simulink model "VTOL_thrust_representation_descent"  (R2020b)
settings: Solver=VariableStepAuto  StartTime=0.0  StopTime=60  RelTol=1e-3
values from neighbouring files (symbols this model uses):
  Aproj = 8.8    [Descent_VTOL_Controller_Design.m]
  Cdvertical = 1    [Descent_VTOL_Controller_Design.m]
  g = 32    [Descent_VTOL_Controller_Design.m]
  Ixx = 13900*lbm2slug/144    (= 2.99236111111)    [Descent_VTOL_Controller_Design.m]
  Ixy = -220*lbm2slug/144    (= -0.0473611111111)    [Descent_VTOL_Controller_Design.m]
  Ixz = -720*lbm2slug/144    (= -0.155)    [Descent_VTOL_Controller_Design.m]
  Iyy = 20150*lbm2slug/144    (= 4.33784722222)    [Descent_VTOL_Controller_Design.m]
  Iyz = -1271*lbm2slug/144    (= -0.273618055556)    [Descent_VTOL_Controller_Design.m]
  Izz = 8300*lbm2slug/144    (= 1.78680555556)    [Descent_VTOL_Controller_Design.m]
  K = lqr(A,B,Q,R)    [Descent_VTOL_Controller_Design.m]
  m = 120*lbm2slug    (= 3.72)    [Descent_VTOL_Controller_Design.m]
  rho = 0.0024    [Descent_VTOL_Controller_Design.m]
  Tbig = 56    [Descent_VTOL_Controller_Design.m]
  Tsmall = 33    [Descent_VTOL_Controller_Design.m]
  xcg1 = (37 - 13.6)/12    (= 1.95)    [Descent_VTOL_Controller_Design.m]
  xcg2 = (44.25 - 37)/12    (= 0.604166666667)    [Descent_VTOL_Controller_Design.m]
undefined symbols (not defined in the file or in its folder): magnitude
libraries: simulink x4, shared6dof x1, aerolibanim x1, dspsigops x1
settings Model: Creator=natha  LastModifiedBy=natha

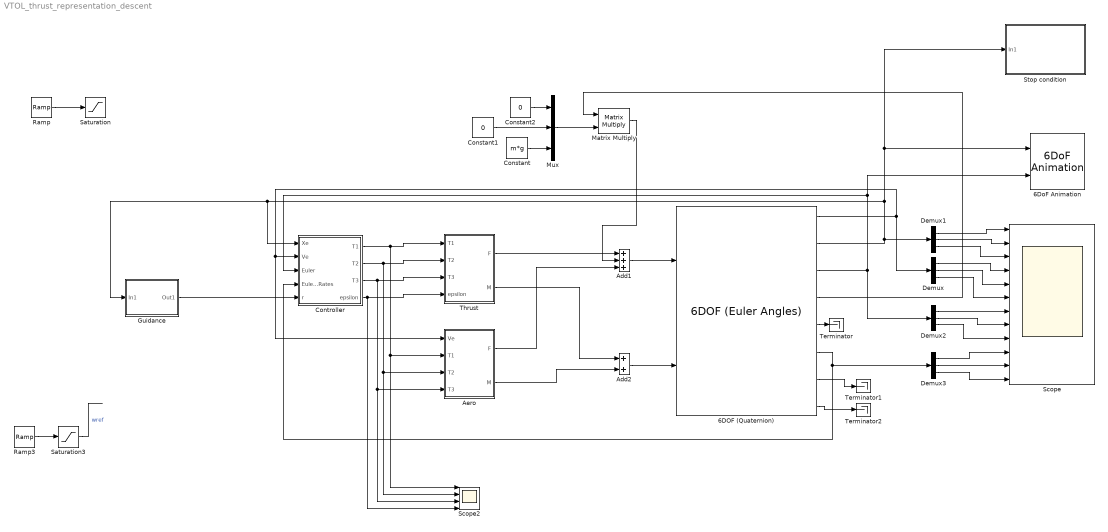
== system VTOL_thrust_representation_descent ==
  6DOF (Quaternion) : shared6dof/6DOF (Euler Angles)  units=Metric (MKS)  mtype=Fixed  rep=Quaternion  xme_0=[0 0 -100]  Vm_0=[0 0 3]  eul_0=[0 0 0]  pm_0=[0 0 0]  mass_0=m  mass_e=0.5  mass_f=2.0  inertia=[Ixx Ixy Ixz; Ixy Iyy Iyz; Ixz Iyz Izz]  inertia_e=eye(3)  inertia_f=2*eye(3)  k_quat=1.0  vre_flag=on  abi_flag=off  aMode=0  xme_statename=''  Vm_statename=''  eul_statename=''  quat_statename=''  pm_statename=''  mass_statename=''
      settings: SourceProductBaseCode=AE,PW,MT,UV,VE,VP
  6DoF Animation : aerolibanim/6DoF Animation  u1=[0 4000 -200 200 -200 200]  u2=0.1  u3=4  u4=[0 0 0]  u5=Fly alongside  u6=[30 100 -30]  u7=10  u8=on
  Add1 : Sum  Inputs=+++
  Add2 : Sum
  Aero : Subsystem
  Constant : Constant  Value=m*g
  Constant1 : Constant  Value=0
  Constant2 : Constant  Value=0
  Controller : Subsystem
  Demux{,1..3} (4 alike) : Demux  Outputs=3
  Guidance : Subsystem
  Matrix Multiply : Product  Multiplication=Matrix(*)
  Mux : Mux  Inputs=3
  Ramp : simulink/Sources/Ramp  slope=-2  start=0  InitialOutput=0
  Ramp3 : simulink/Sources/Ramp  slope=-1  start=0  InitialOutput=0
  Saturation : Saturate  UpperLimit=0  LowerLimit=-5  LinearizeAsGain=off
  Saturation3 : Saturate  UpperLimit=3  LowerLimit=0.5  LinearizeAsGain=off
  Scope : Scope  NumInputPorts=12
  Scope2 : Scope  NumInputPorts=4
  Stop condition : Subsystem
  Terminator : Terminator
  Terminator1 : Terminator
  Terminator2 : Terminator
  Thrust : Subsystem
  wires:
  Demux/2 -> Scope/5
  Demux2/3 -> Scope/9
  Demux3/1 -> Scope/10
  Demux/1 -> Scope/4
  Demux2/2 -> Scope/8
  Demux1/2 -> Scope/2
  Demux1/1 -> Scope/1
  Thrust/1(F) -> Add1/1
  Constant1/1 -> Mux/2
  Matrix Multiply/1 -> Add1/2
  Mux/1 -> Matrix Multiply/2
  Add1/1 -> 6DOF (Quaternion)/1
  Demux/3 -> Scope/6
  6DOF (Quaternion)/3 -> Demux2/1, 6DoF Animation/2, Controller/3(Euler)
  6DOF (Quaternion)/1 -> Demux/1, Aero/1(Ve), Controller/2(Ve)
  Demux3/3 -> Scope/12
  Demux2/1 -> Scope/7
  6DOF (Quaternion)/4 -> Matrix Multiply/1
  6DOF (Quaternion)/2 -> Demux1/1, Stop condition/1(In1), 6DoF Animation/1, Guidance/1(In1), Controller/1(Xe)
  Demux1/3 -> Scope/3
  Demux3/2 -> Scope/11
  Constant2/1 -> Mux/1
  Constant/1 -> Mux/3
  6DOF (Quaternion)/6 -> Demux3/1, Controller/4(Euler Rates)
  Controller/4(epsilon) -> Thrust/4(epsilon), Scope2/4
  Controller/2(T2) -> Aero/3(T2), Scope2/2, Thrust/2(T2)
  Controller/3(T3) -> Aero/4(T3), Scope2/3, Thrust/3(T3)
  Controller/1(T1) -> Aero/2(T1), Scope2/1, Thrust/1(T1)
  Add2/1 -> 6DOF (Quaternion)/2
  Aero/2(M) -> Add2/2
  Thrust/2(M) -> Add2/1
  Aero/1(F) -> Add1/3
  Ramp/1 -> Saturation/1
  6DOF (Quaternion)/5 -> Terminator/1
  6DOF (Quaternion)/7 -> Terminator1/1
  6DOF (Quaternion)/8 -> Terminator2/1
  Ramp3/1 -> Saturation3/1
  Saturation3/1 -> ?  "wref"
  Guidance/1(Out1) -> Controller/5(r)

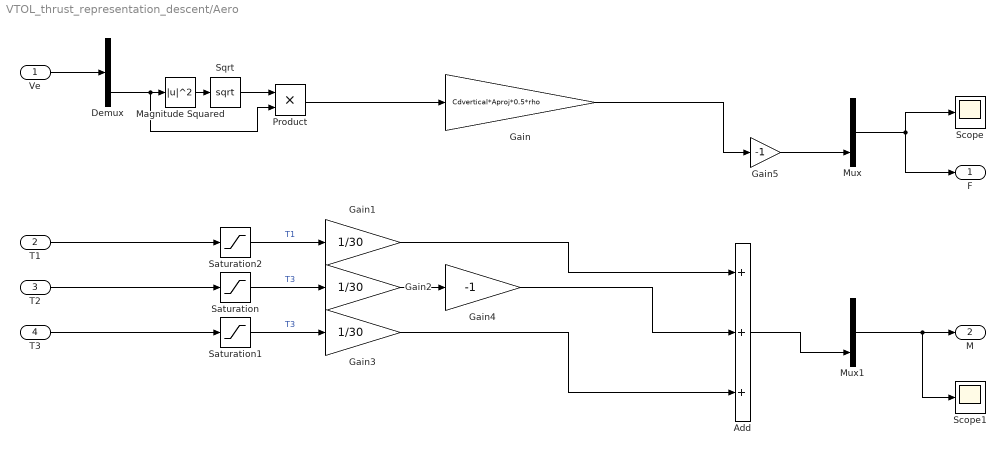
== system VTOL_thrust_representation_descent/Aero ==
  Ve : Inport
  T1 : Inport  Port=2
  T2 : Inport  Port=3
  T3 : Inport  Port=4
  Add : Sum  Inputs=+++
  Demux : Demux  Outputs=3
  Gain : Gain  Gain=Cdvertical*Aproj*0.5*rho
  Gain1 : Gain  Gain=1/30
  Gain2 : Gain  Gain=1/30
  Gain3 : Gain  Gain=1/30
  Gain4 : Gain  Gain=-1
  Gain5 : Gain  Gain=-1
  Magnitude Squared : Math  Operator=magnitude^2  SaturateOnIntegerOverflow=on
  Mux : Mux  Inputs=3
  Mux1 : Mux  Inputs=3
  Product : Product
  Saturation : Saturate  UpperLimit=Tbig  LowerLimit=0
  Saturation1 : Saturate  UpperLimit=Tbig  LowerLimit=0
  Saturation2 : Saturate  UpperLimit=Tsmall  LowerLimit=0
  Scope : Scope
  Scope1 : Scope
  Sqrt : Sqrt  SaturateOnIntegerOverflow=on
  F : Outport
  M : Outport  Port=2
  wires:
  Ve/1 -> Demux/1
  Demux/3 -> Product/2, Magnitude Squared/1
  Magnitude Squared/1 -> Sqrt/1
  Sqrt/1 -> Product/1
  Product/1 -> Gain/1
  Mux/1 -> Scope/1, F/1
  Gain/1 -> Gain5/1
  T3/1 -> Saturation1/1
  T2/1 -> Saturation/1
  T1/1 -> Saturation2/1
  Saturation2/1 -> Gain1/1  "T1"
  Mux1/1 -> Scope1/1, M/1
  Saturation/1 -> Gain2/1  "T3"
  Saturation1/1 -> Gain3/1  "T3"
  Add/1 -> Mux1/3
  Gain3/1 -> Add/3
  Gain2/1 -> Gain4/1
  Gain1/1 -> Add/1
  Gain4/1 -> Add/2
  Gain5/1 -> Mux/3

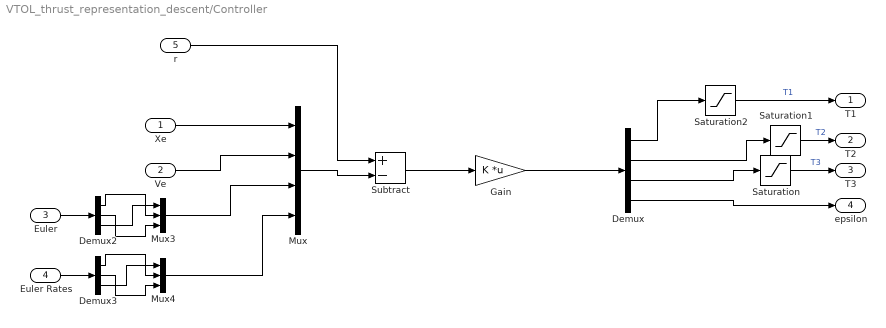
== system VTOL_thrust_representation_descent/Controller ==
  Xe : Inport
  Ve : Inport  Port=2
  Euler : Inport  Port=3
  Euler Rates : Inport  Port=4
  r : Inport  Port=5
  Demux : Demux
  Demux2 : Demux  Outputs=3
  Demux3 : Demux  Outputs=3
  Gain : Gain  Gain=K  Multiplication=Matrix(K*u)
  Mux : Mux
  Mux3 : Mux  Inputs=3
  Mux4 : Mux  Inputs=3
  Saturation : Saturate  UpperLimit=Tbig  LowerLimit=0
  Saturation1 : Saturate  UpperLimit=Tbig  LowerLimit=0
  Saturation2 : Saturate  UpperLimit=Tsmall  LowerLimit=0
  Subtract : Sum  Inputs=+-
  T1 : Outport
  T2 : Outport  Port=2
  T3 : Outport  Port=3
  epsilon : Outport  Port=4
  wires:
  Xe/1 -> Mux/1
  Ve/1 -> Mux/2
  Gain/1 -> Demux/1
  Demux/4 -> epsilon/1
  r/1 -> Subtract/1
  Mux/1 -> Subtract/2
  Subtract/1 -> Gain/1
  Euler/1 -> Demux2/1
  Euler Rates/1 -> Demux3/1
  Demux2/1 -> Mux3/2
  Demux2/2 -> Mux3/3
  Demux2/3 -> Mux3/1
  Demux3/1 -> Mux4/2
  Demux3/2 -> Mux4/3
  Demux3/3 -> Mux4/1
  Mux3/1 -> Mux/3
  Mux4/1 -> Mux/4
  Demux/3 -> Saturation/1
  Demux/2 -> Saturation1/1
  Demux/1 -> Saturation2/1
  Saturation/1 -> T3/1  "T3"
  Saturation1/1 -> T2/1  "T2"
  Saturation2/1 -> T1/1  "T1"

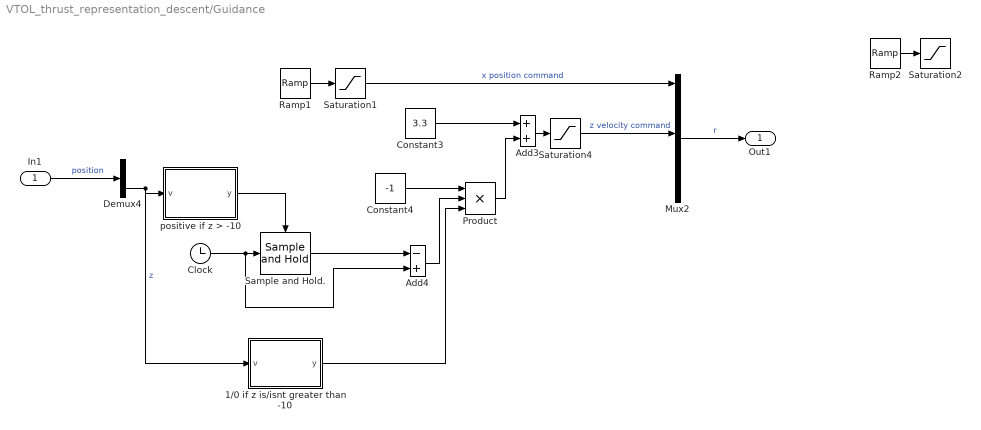
== system VTOL_thrust_representation_descent/Guidance ==
  In1 : Inport
  1/0 if z is/isnt greater than -10 : MATLAB Function  TreatAsAtomicUnit=on
  Add3 : Sum
  Add4 : Sum  Inputs=-+
  Clock : Clock
  Constant3 : Constant  Value=3.3
  Constant4 : Constant  Value=-1
  Demux4 : Demux  Outputs=3
  Mux2 : Mux  Inputs=12
  Product : Product  Inputs=3
  Ramp1 : simulink/Sources/Ramp  slope=4  start=0  InitialOutput=0
  Ramp2 : simulink/Sources/Ramp  slope=1  start=0  InitialOutput=0
  Sample and Hold. : dspsigops/Sample and Hold  trig=Rising edge  initCond=0  latchinput=off
  Saturation1 : Saturate  UpperLimit=100  LowerLimit=0  LinearizeAsGain=off
  Saturation2 : Saturate  UpperLimit=0  LowerLimit=0  LinearizeAsGain=off
  Saturation4 : Saturate  UpperLimit=3  LowerLimit=0.5
  positive if z > -10 : MATLAB Function  TreatAsAtomicUnit=on
  Out1 : Outport
  wires:
  Demux4/3 -> positive if z > -10/1(v), 1/0 if z is/isnt greater than -10/1(v)  "z"
  Clock/1 -> Add4/2, Sample and Hold./1
  1/0 if z is/isnt greater than -10/1(y) -> Product/3
  Saturation4/1 -> Mux2/6  "z velocity command"
  Ramp1/1 -> Saturation1/1
  Sample and Hold./1 -> Add4/1
  Ramp2/1 -> Saturation2/1
  Saturation1/1 -> Mux2/1  "x position command"
  Product/1 -> Add3/2
  In1/1 -> Demux4/1  "position"
  Add4/1 -> Product/2
  Add3/1 -> Saturation4/1
  Constant3/1 -> Add3/1
  Constant4/1 -> Product/1
  positive if z > -10/1(y) -> Sample and Hold./Trigger
  Mux2/1 -> Out1/1  "r"

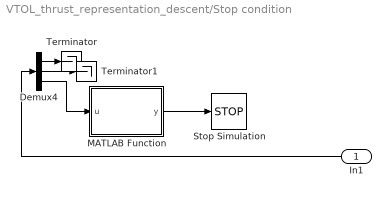
== system VTOL_thrust_representation_descent/Stop condition ==
  In1 : Inport
  Demux4 : Demux  Outputs=3
  MATLAB Function : MATLAB Function  TreatAsAtomicUnit=on
  Stop Simulation : Stop
  Terminator : Terminator
  Terminator1 : Terminator
  wires:
  MATLAB Function/1(y) -> Stop Simulation/1
  Demux4/3 -> MATLAB Function/1(u)
  In1/1 -> Demux4/1
  Demux4/2 -> Terminator1/1
  Demux4/1 -> Terminator/1

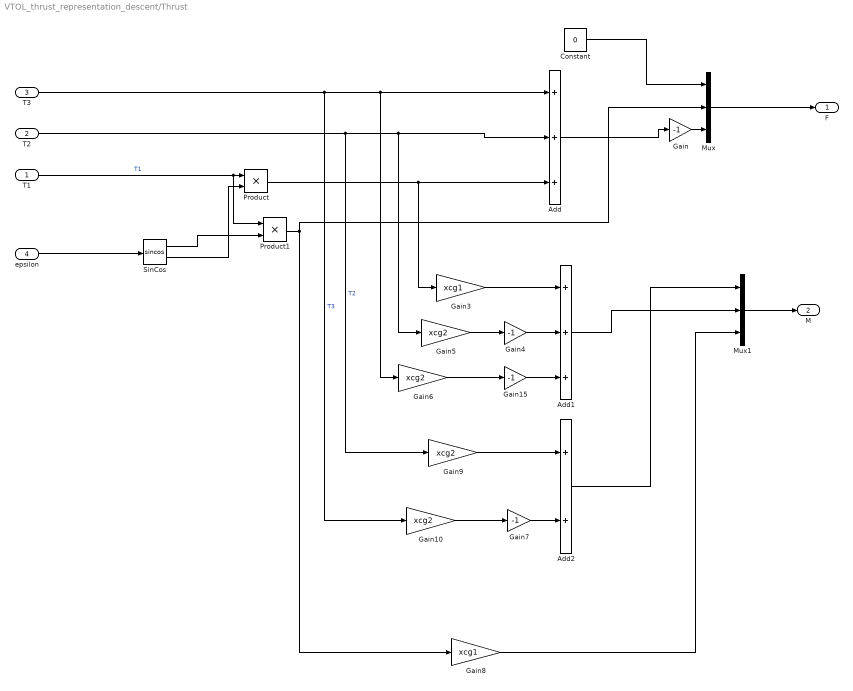
== system VTOL_thrust_representation_descent/Thrust ==
  T1 : Inport
  T2 : Inport  Port=2
  T3 : Inport  Port=3
  epsilon : Inport  Port=4
  Add : Sum  Inputs=+++
  Add1 : Sum  Inputs=+++
  Add2 : Sum
  Constant : Constant  Value=0
  Gain{,4,7,15} (4 alike) : Gain  Gain=-1
  Gain{5..6,9..10} (4 alike) : Gain  Gain=xcg2
  Gain3 : Gain  Gain=xcg1
  Gain8 : Gain  Gain=xcg1
  Mux : Mux  Inputs=3
  Mux1 : Mux  Inputs=3
  Product : Product
  Product1 : Product
  SinCos : Trigonometry  Operator=sincos
  F : Outport
  M : Outport  Port=2
  wires:
  SinCos/1 -> Product1/2
  Product/1 -> Add/3, Gain3/1
  T1/1 -> Product1/1, Product/1  "T1"
  SinCos/2 -> Product/2
  Mux/1 -> F/1
  epsilon/1 -> SinCos/1
  Mux1/1 -> M/1
  Gain3/1 -> Add1/1
  Gain5/1 -> Gain4/1
  Gain6/1 -> Gain15/1
  T3/1 -> Gain10/1, Add/1, Gain6/1  "T3"
  T2/1 -> Gain9/1, Add/2, Gain5/1  "T2"
  Gain9/1 -> Add2/1
  Gain10/1 -> Gain7/1
  Add2/1 -> Mux1/1
  Gain7/1 -> Add2/2
  Constant/1 -> Mux/1
  Product1/1 -> Mux/2, Gain8/1
  Add1/1 -> Mux1/2
  Gain8/1 -> Mux1/3
  Gain4/1 -> Add1/2
  Gain15/1 -> Add1/3
  Add/1 -> Gain/1
  Gain/1 -> Mux/3

== matlab function VTOL_thrust_representation_descent/Stop condition/MATLAB Function ==
  data: u input; y output
function y = fcn(u)
stop = 0;
if u > 0
    stop = 1;
end
y = stop;

== matlab function VTOL_thrust_representation_descent/Guidance/1//0 if z is//isnt greater than -10 ==
  data: v input; y output
function y = fcn(v)
out = 0;
if v > -10
    out = 1;
end

y = out;

== matlab function VTOL_thrust_representation_descent/Guidance/positive if z > -10 ==
  data: v input; y output
function y = fcn(v)

out = v + 10;

y = out;
